simulink model "RelayZN_BlueRVO2_Control"  (R2023b)
settings: Solver=FixedStepAuto  StartTime=0.0  StopTime=600  FixedStep=0.01  RelTol=1e-3
values from neighbouring files (symbols this model uses):
  Kd_heave = 0.0666*Kc*Tc    (= 4.43668844611)    [RelayTest_controllerCalc.m]
  Kd_pitch = 0.0666*Kc*Tc    (= 1.01222543806)    [RelayTest_controllerCalc.m]
  Kd_roll = 0.0666*Kc*Tc    (= 0.877495471431)    [RelayTest_controllerCalc.m]
  Kd_surge = 0.0666*Kc*Tc    (= 11.6366264628)    [RelayTest_controllerCalc.m]
  Kd_sway = 0.0666*Kc*Tc    (= 3.84334224278)    [RelayTest_controllerCalc.m]
  Kd_yaw = 0.0666*Kc*Tc    (= 0.976135030348)    [RelayTest_controllerCalc.m]
  Ki_heave = 0.4*Kc/Tc    (= 0.123145727686)    [RelayTest_controllerCalc.m]
  Ki_pitch = 0.4*Kc/Tc    (= 0.865707662577)    [RelayTest_controllerCalc.m]
  Ki_roll = 0.4*Kc/Tc    (= 0.00801668103365)    [RelayTest_controllerCalc.m]
  Ki_surge = 0.4*Kc/Tc    (= 0.186852931714)    [RelayTest_controllerCalc.m]
  Ki_sway = 0.4*Kc/Tc    (= 0.0254608741636)    [RelayTest_controllerCalc.m]
  Ki_yaw = 0.4*Kc/Tc    (= 0.0110729266567)    [RelayTest_controllerCalc.m]
  Kp_heave = 0.2*Kc    (= 0.905736827128)    [RelayTest_controllerCalc.m]
  Kp_pitch = 0.2*Kc    (= 1.14706265291)    [RelayTest_controllerCalc.m]
  Kp_roll = 0.2*Kc    (= 0.102773850851)    [RelayTest_controllerCalc.m]
  Kp_surge = 0.2*Kc    (= 1.80686784967)    [RelayTest_controllerCalc.m]
  Kp_yaw = 0.2*Kc    (= 0.127394021185)    [RelayTest_controllerCalc.m]
libraries: slpidlib x18
(part 2 of 2)

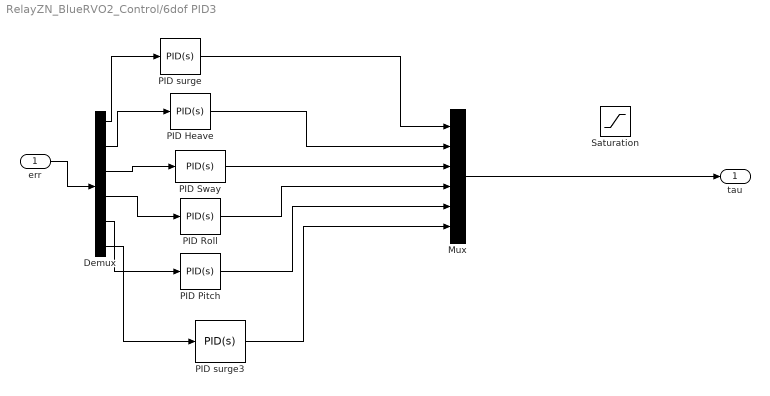
== system RelayZN_BlueRVO2_Control/6dof PID3 ==
  err : Inport
  Demux : Demux  Outputs=6
  Mux : Mux  Inputs=6
  PID Heave : slpidlib/PID Controller  Controller=PID  Form=Parallel  TimeDomain=Continuous-time  UseExternalTs=off  SampleTime=-1  IntegratorMethod=Forward Euler  FilterMethod=Forward Euler  ControllerParametersSource=internal  P=120  I=203  UseKiTs=off  D=17.7  N=100  UseFilter=on  TunerSelectOption=Transfer Function Based (PID Tuner App)  InitialConditionSource=internal  InitialConditionForIntegrator=0  InitialConditionForFilter=0  DifferentiatorICPrevScaledInput=0  ExternalReset=none  TrackingMode=off  Kt=1  LimitOutput=off  SatLimitsSource=internal  UpperSaturationLimit=inf  LowerSaturationLimit=-inf  LinearizeAsGain=on  AntiWindupMode=none  Kb=1  LimitIntegrator=off  UpperIntegratorSaturationLimit=inf  LowerIntegratorSaturationLimit=-inf  POutMin=[]  POutMax=[]  IOutMin=[]  IOutMax=[]  DOutMin=[]  DOutMax=[]  NOutMin=[]  NOutMax=[]  SumOutMin=[]  SumOutMax=[]  SaturationOutMin=[]  SaturationOutMax=[]  PParamMin=[]  PParamMax=[]  IParamMin=[]  IParamMax=[]  DParamMin=[]  DParamMax=[]  NParamMin=[]  NParamMax=[]  KbParamMin=[]  KbParamMax=[]  KtParamMin=[]  KtParamMax=[]  KbOutMin=[]  KbOutMax=[]  KtOutMin=[]  KtOutMax=[]  IntegratorOutMin=[]  IntegratorOutMax=[]  FilterOutMin=[]  FilterOutMax=[]  SumI1OutMin=[]  SumI1OutMax=[]  SumI2OutMin=[]  SumI2OutMax=[]  SumI3OutMin=[]  SumI3OutMax=[]  SumI4OutMin=[]  SumI4OutMax=[]  SumDOutMin=[]  SumDOutMax=[]  DifferentiatorOutMin=[]  DifferentiatorOutMax=[]  FilterDiffOutCoefMin=[]  FilterDiffOutCoefMax=[]  ReciprocalOutMin=[]  ReciprocalOutMax=[]  SumDenOutMin=[]  SumDenOutMax=[]  SumNumOutMin=[]  SumNumOutMax=[]  DivideOutMin=[]  DivideOutMax=[]  UdiffTsProdOutMin=[]  UdiffTsProdOutMax=[]  NTsProdOutMin=[]  NTsProdOutMax=[]  UintegralTsProdOutMin=[]  UintegralTsProdOutMax=[]  UngainTsProdOutMin=[]  UngainTsProdOutMax=[]  ClampingZeroOutDataTypeStr=Inherit: Inherit via back propagation  ClampingZeroOutMin=[]  ClampingZeroOutMax=[]  FilterDenConstantOutDataTypeStr=Inherit: Inherit via back propagation  FilterDenConstantOutMin=[]  FilterDenConstantOutMax=[]  PCopyOutDataTypeStr=Inherit: Inherit via back propagation  PCopyOutMin=[]  PCopyOutMax=[]  NCopyOutDataTypeStr=Inherit: Inherit via back propagation  NCopyOutMin=[]  NCopyOutMax=[]  IntegratorContinuousStateAttributes=''  IntegratorStateMustResolveToSignalObject=off  IntegratorRTWStateStorageClass=Auto  FilterContinuousStateAttributes=''  FilterStateMustResolveToSignalObject=off  FilterRTWStateStorageClass=Auto  ParallelPVariant=InternalParameters  IdealPVariant=Disabled  IVariant=InternalParameters  DVariant=InternalParameters  IntegratorVariant=Continuous  SatVariant=Disabled  AWVariant=Passthrough  PCopyVariant=Disabled  TRVariant=Disabled  FdbkBlocksVariant=Forward  IdealPFdbkVariant=Disabled  SatFdbkVariant=Disabled  DerivativeFilterVariant=ContFilter  NVariant=InternalParameters  NCopyVariant=Disabled  FilterICVariant=InternalICsFilter  IntegratorICVariant=InternalICs  ExternalResetVariant=Disabled  TRSumVariant=Passthrough  SumFdbkVariant=Disabled  SumVariant=Sum_PID  TsampFilterVariant=InternalTs  TsampNgainVariant=Passthrough  TsampIntegralVariant=Disabled_SignalSpec  ExternalSaturationOutDataTypeStr=Inherit: Same as second input
  PID Pitch : slpidlib/PID Controller  Controller=PID  Form=Parallel  TimeDomain=Continuous-time  UseExternalTs=off  SampleTime=-1  IntegratorMethod=Forward Euler  FilterMethod=Forward Euler  ControllerParametersSource=internal  P=4.2  I=8.4  UseKiTs=off  D=0.525  N=100  UseFilter=on  TunerSelectOption=Transfer Function Based (PID Tuner App)  InitialConditionSource=internal  InitialConditionForIntegrator=0  InitialConditionForFilter=0  DifferentiatorICPrevScaledInput=0  ExternalReset=none  TrackingMode=off  Kt=1  LimitOutput=off  SatLimitsSource=internal  UpperSaturationLimit=inf  LowerSaturationLimit=-inf  LinearizeAsGain=on  AntiWindupMode=none  Kb=1  LimitIntegrator=off  UpperIntegratorSaturationLimit=inf  LowerIntegratorSaturationLimit=-inf  POutMin=[]  POutMax=[]  IOutMin=[]  IOutMax=[]  DOutMin=[]  DOutMax=[]  NOutMin=[]  NOutMax=[]  SumOutMin=[]  SumOutMax=[]  SaturationOutMin=[]  SaturationOutMax=[]  PParamMin=[]  PParamMax=[]  IParamMin=[]  IParamMax=[]  DParamMin=[]  DParamMax=[]  NParamMin=[]  NParamMax=[]  KbParamMin=[]  KbParamMax=[]  KtParamMin=[]  KtParamMax=[]  KbOutMin=[]  KbOutMax=[]  KtOutMin=[]  KtOutMax=[]  IntegratorOutMin=[]  IntegratorOutMax=[]  FilterOutMin=[]  FilterOutMax=[]  SumI1OutMin=[]  SumI1OutMax=[]  SumI2OutMin=[]  SumI2OutMax=[]  SumI3OutMin=[]  SumI3OutMax=[]  SumI4OutMin=[]  SumI4OutMax=[]  SumDOutMin=[]  SumDOutMax=[]  DifferentiatorOutMin=[]  DifferentiatorOutMax=[]  FilterDiffOutCoefMin=[]  FilterDiffOutCoefMax=[]  ReciprocalOutMin=[]  ReciprocalOutMax=[]  SumDenOutMin=[]  SumDenOutMax=[]  SumNumOutMin=[]  SumNumOutMax=[]  DivideOutMin=[]  DivideOutMax=[]  UdiffTsProdOutMin=[]  UdiffTsProdOutMax=[]  NTsProdOutMin=[]  NTsProdOutMax=[]  UintegralTsProdOutMin=[]  UintegralTsProdOutMax=[]  UngainTsProdOutMin=[]  UngainTsProdOutMax=[]  ClampingZeroOutDataTypeStr=Inherit: Inherit via back propagation  ClampingZeroOutMin=[]  ClampingZeroOutMax=[]  FilterDenConstantOutDataTypeStr=Inherit: Inherit via back propagation  FilterDenConstantOutMin=[]  FilterDenConstantOutMax=[]  PCopyOutDataTypeStr=Inherit: Inherit via back propagation  PCopyOutMin=[]  PCopyOutMax=[]  NCopyOutDataTypeStr=Inherit: Inherit via back propagation  NCopyOutMin=[]  NCopyOutMax=[]  IntegratorContinuousStateAttributes=''  IntegratorStateMustResolveToSignalObject=off  IntegratorRTWStateStorageClass=Auto  FilterContinuousStateAttributes=''  FilterStateMustResolveToSignalObject=off  FilterRTWStateStorageClass=Auto  ParallelPVariant=InternalParameters  IdealPVariant=Disabled  IVariant=InternalParameters  DVariant=InternalParameters  IntegratorVariant=Continuous  SatVariant=Disabled  AWVariant=Passthrough  PCopyVariant=Disabled  TRVariant=Disabled  FdbkBlocksVariant=Forward  IdealPFdbkVariant=Disabled  SatFdbkVariant=Disabled  DerivativeFilterVariant=ContFilter  NVariant=InternalParameters  NCopyVariant=Disabled  FilterICVariant=InternalICsFilter  IntegratorICVariant=InternalICs  ExternalResetVariant=Disabled  TRSumVariant=Passthrough  SumFdbkVariant=Disabled  SumVariant=Sum_PID  TsampFilterVariant=InternalTs  TsampNgainVariant=Passthrough  TsampIntegralVariant=Disabled_SignalSpec  ExternalSaturationOutDataTypeStr=Inherit: Same as second input
  PID Roll : slpidlib/PID Controller  Controller=PID  Form=Parallel  TimeDomain=Continuous-time  UseExternalTs=off  SampleTime=-1  IntegratorMethod=Forward Euler  FilterMethod=Forward Euler  ControllerParametersSource=internal  P=3.6  I=6.37  UseKiTs=off  D=0.51  N=100  UseFilter=on  TunerSelectOption=Transfer Function Based (PID Tuner App)  InitialConditionSource=internal  InitialConditionForIntegrator=0  InitialConditionForFilter=0  DifferentiatorICPrevScaledInput=0  ExternalReset=none  TrackingMode=off  Kt=1  LimitOutput=off  SatLimitsSource=internal  UpperSaturationLimit=inf  LowerSaturationLimit=-inf  LinearizeAsGain=on  AntiWindupMode=none  Kb=1  LimitIntegrator=off  UpperIntegratorSaturationLimit=inf  LowerIntegratorSaturationLimit=-inf  POutMin=[]  POutMax=[]  IOutMin=[]  IOutMax=[]  DOutMin=[]  DOutMax=[]  NOutMin=[]  NOutMax=[]  SumOutMin=[]  SumOutMax=[]  SaturationOutMin=[]  SaturationOutMax=[]  PParamMin=[]  PParamMax=[]  IParamMin=[]  IParamMax=[]  DParamMin=[]  DParamMax=[]  NParamMin=[]  NParamMax=[]  KbParamMin=[]  KbParamMax=[]  KtParamMin=[]  KtParamMax=[]  KbOutMin=[]  KbOutMax=[]  KtOutMin=[]  KtOutMax=[]  IntegratorOutMin=[]  IntegratorOutMax=[]  FilterOutMin=[]  FilterOutMax=[]  SumI1OutMin=[]  SumI1OutMax=[]  SumI2OutMin=[]  SumI2OutMax=[]  SumI3OutMin=[]  SumI3OutMax=[]  SumI4OutMin=[]  SumI4OutMax=[]  SumDOutMin=[]  SumDOutMax=[]  DifferentiatorOutMin=[]  DifferentiatorOutMax=[]  FilterDiffOutCoefMin=[]  FilterDiffOutCoefMax=[]  ReciprocalOutMin=[]  ReciprocalOutMax=[]  SumDenOutMin=[]  SumDenOutMax=[]  SumNumOutMin=[]  SumNumOutMax=[]  DivideOutMin=[]  DivideOutMax=[]  UdiffTsProdOutMin=[]  UdiffTsProdOutMax=[]  NTsProdOutMin=[]  NTsProdOutMax=[]  UintegralTsProdOutMin=[]  UintegralTsProdOutMax=[]  UngainTsProdOutMin=[]  UngainTsProdOutMax=[]  ClampingZeroOutDataTypeStr=Inherit: Inherit via back propagation  ClampingZeroOutMin=[]  ClampingZeroOutMax=[]  FilterDenConstantOutDataTypeStr=Inherit: Inherit via back propagation  FilterDenConstantOutMin=[]  FilterDenConstantOutMax=[]  PCopyOutDataTypeStr=Inherit: Inherit via back propagation  PCopyOutMin=[]  PCopyOutMax=[]  NCopyOutDataTypeStr=Inherit: Inherit via back propagation  NCopyOutMin=[]  NCopyOutMax=[]  IntegratorContinuousStateAttributes=''  IntegratorStateMustResolveToSignalObject=off  IntegratorRTWStateStorageClass=Auto  FilterContinuousStateAttributes=''  FilterStateMustResolveToSignalObject=off  FilterRTWStateStorageClass=Auto  ParallelPVariant=InternalParameters  IdealPVariant=Disabled  IVariant=InternalParameters  DVariant=InternalParameters  IntegratorVariant=Continuous  SatVariant=Disabled  AWVariant=Passthrough  PCopyVariant=Disabled  TRVariant=Disabled  FdbkBlocksVariant=Forward  IdealPFdbkVariant=Disabled  SatFdbkVariant=Disabled  DerivativeFilterVariant=ContFilter  NVariant=InternalParameters  NCopyVariant=Disabled  FilterICVariant=InternalICsFilter  IntegratorICVariant=InternalICs  ExternalResetVariant=Disabled  TRSumVariant=Passthrough  SumFdbkVariant=Disabled  SumVariant=Sum_PID  TsampFilterVariant=InternalTs  TsampNgainVariant=Passthrough  TsampIntegralVariant=Disabled_SignalSpec  ExternalSaturationOutDataTypeStr=Inherit: Same as second input
  PID Sway : slpidlib/PID Controller  Controller=PID  Form=Parallel  TimeDomain=Continuous-time  UseExternalTs=off  SampleTime=-1  IntegratorMethod=Forward Euler  FilterMethod=Forward Euler  ControllerParametersSource=internal  P=120  I=208.7  UseKiTs=off  D=17.25  N=100  UseFilter=on  TunerSelectOption=Transfer Function Based (PID Tuner App)  InitialConditionSource=internal  InitialConditionForIntegrator=5  InitialConditionForFilter=0  DifferentiatorICPrevScaledInput=0  ExternalReset=none  TrackingMode=off  Kt=1  LimitOutput=off  SatLimitsSource=internal  UpperSaturationLimit=inf  LowerSaturationLimit=-inf  LinearizeAsGain=on  AntiWindupMode=none  Kb=1  LimitIntegrator=off  UpperIntegratorSaturationLimit=inf  LowerIntegratorSaturationLimit=-inf  POutMin=[]  POutMax=[]  IOutMin=[]  IOutMax=[]  DOutMin=[]  DOutMax=[]  NOutMin=[]  NOutMax=[]  SumOutMin=[]  SumOutMax=[]  SaturationOutMin=[]  SaturationOutMax=[]  PParamMin=[]  PParamMax=[]  IParamMin=[]  IParamMax=[]  DParamMin=[]  DParamMax=[]  NParamMin=[]  NParamMax=[]  KbParamMin=[]  KbParamMax=[]  KtParamMin=[]  KtParamMax=[]  KbOutMin=[]  KbOutMax=[]  KtOutMin=[]  KtOutMax=[]  IntegratorOutMin=[]  IntegratorOutMax=[]  FilterOutMin=[]  FilterOutMax=[]  SumI1OutMin=[]  SumI1OutMax=[]  SumI2OutMin=[]  SumI2OutMax=[]  SumI3OutMin=[]  SumI3OutMax=[]  SumI4OutMin=[]  SumI4OutMax=[]  SumDOutMin=[]  SumDOutMax=[]  DifferentiatorOutMin=[]  DifferentiatorOutMax=[]  FilterDiffOutCoefMin=[]  FilterDiffOutCoefMax=[]  ReciprocalOutMin=[]  ReciprocalOutMax=[]  SumDenOutMin=[]  SumDenOutMax=[]  SumNumOutMin=[]  SumNumOutMax=[]  DivideOutMin=[]  DivideOutMax=[]  UdiffTsProdOutMin=[]  UdiffTsProdOutMax=[]  NTsProdOutMin=[]  NTsProdOutMax=[]  UintegralTsProdOutMin=[]  UintegralTsProdOutMax=[]  UngainTsProdOutMin=[]  UngainTsProdOutMax=[]  ClampingZeroOutDataTypeStr=Inherit: Inherit via back propagation  ClampingZeroOutMin=[]  ClampingZeroOutMax=[]  FilterDenConstantOutDataTypeStr=Inherit: Inherit via back propagation  FilterDenConstantOutMin=[]  FilterDenConstantOutMax=[]  PCopyOutDataTypeStr=Inherit: Inherit via back propagation  PCopyOutMin=[]  PCopyOutMax=[]  NCopyOutDataTypeStr=Inherit: Inherit via back propagation  NCopyOutMin=[]  NCopyOutMax=[]  IntegratorContinuousStateAttributes=''  IntegratorStateMustResolveToSignalObject=off  IntegratorRTWStateStorageClass=Auto  FilterContinuousStateAttributes=''  FilterStateMustResolveToSignalObject=off  FilterRTWStateStorageClass=Auto  ParallelPVariant=InternalParameters  IdealPVariant=Disabled  IVariant=InternalParameters  DVariant=InternalParameters  IntegratorVariant=Continuous  SatVariant=Disabled  AWVariant=Passthrough  PCopyVariant=Disabled  TRVariant=Disabled  FdbkBlocksVariant=Forward  IdealPFdbkVariant=Disabled  SatFdbkVariant=Disabled  DerivativeFilterVariant=ContFilter  NVariant=InternalParameters  NCopyVariant=Disabled  FilterICVariant=InternalICsFilter  IntegratorICVariant=InternalICs  ExternalResetVariant=Disabled  TRSumVariant=Passthrough  SumFdbkVariant=Disabled  SumVariant=Sum_PID  TsampFilterVariant=InternalTs  TsampNgainVariant=Passthrough  TsampIntegralVariant=Disabled_SignalSpec  ExternalSaturationOutDataTypeStr=Inherit: Same as second input
  PID surge : slpidlib/PID Controller  Controller=PID  Form=Parallel  TimeDomain=Continuous-time  UseExternalTs=off  SampleTime=-1  IntegratorMethod=Forward Euler  FilterMethod=Forward Euler  ControllerParametersSource=internal  P=3.06  I=0.57  UseKiTs=off  D=4.1  N=100  UseFilter=on  TunerSelectOption=Transfer Function Based (PID Tuner App)  InitialConditionSource=internal  InitialConditionForIntegrator=0  InitialConditionForFilter=0  DifferentiatorICPrevScaledInput=0  ExternalReset=none  TrackingMode=off  Kt=1  LimitOutput=off  SatLimitsSource=internal  UpperSaturationLimit=inf  LowerSaturationLimit=-inf  LinearizeAsGain=on  AntiWindupMode=none  Kb=1  LimitIntegrator=off  UpperIntegratorSaturationLimit=inf  LowerIntegratorSaturationLimit=-inf  POutMin=[]  POutMax=[]  IOutMin=[]  IOutMax=[]  DOutMin=[]  DOutMax=[]  NOutMin=[]  NOutMax=[]  SumOutMin=[]  SumOutMax=[]  SaturationOutMin=[]  SaturationOutMax=[]  PParamMin=[]  PParamMax=[]  IParamMin=[]  IParamMax=[]  DParamMin=[]  DParamMax=[]  NParamMin=[]  NParamMax=[]  KbParamMin=[]  KbParamMax=[]  KtParamMin=[]  KtParamMax=[]  KbOutMin=[]  KbOutMax=[]  KtOutMin=[]  KtOutMax=[]  IntegratorOutMin=[]  IntegratorOutMax=[]  FilterOutMin=[]  FilterOutMax=[]  SumI1OutMin=[]  SumI1OutMax=[]  SumI2OutMin=[]  SumI2OutMax=[]  SumI3OutMin=[]  SumI3OutMax=[]  SumI4OutMin=[]  SumI4OutMax=[]  SumDOutMin=[]  SumDOutMax=[]  DifferentiatorOutMin=[]  DifferentiatorOutMax=[]  FilterDiffOutCoefMin=[]  FilterDiffOutCoefMax=[]  ReciprocalOutMin=[]  ReciprocalOutMax=[]  SumDenOutMin=[]  SumDenOutMax=[]  SumNumOutMin=[]  SumNumOutMax=[]  DivideOutMin=[]  DivideOutMax=[]  UdiffTsProdOutMin=[]  UdiffTsProdOutMax=[]  NTsProdOutMin=[]  NTsProdOutMax=[]  UintegralTsProdOutMin=[]  UintegralTsProdOutMax=[]  UngainTsProdOutMin=[]  UngainTsProdOutMax=[]  ClampingZeroOutDataTypeStr=Inherit: Inherit via back propagation  ClampingZeroOutMin=[]  ClampingZeroOutMax=[]  FilterDenConstantOutDataTypeStr=Inherit: Inherit via back propagation  FilterDenConstantOutMin=[]  FilterDenConstantOutMax=[]  PCopyOutDataTypeStr=Inherit: Inherit via back propagation  PCopyOutMin=[]  PCopyOutMax=[]  NCopyOutDataTypeStr=Inherit: Inherit via back propagation  NCopyOutMin=[]  NCopyOutMax=[]  IntegratorContinuousStateAttributes=''  IntegratorStateMustResolveToSignalObject=off  IntegratorRTWStateStorageClass=Auto  FilterContinuousStateAttributes=''  FilterStateMustResolveToSignalObject=off  FilterRTWStateStorageClass=Auto  ParallelPVariant=InternalParameters  IdealPVariant=Disabled  IVariant=InternalParameters  DVariant=InternalParameters  IntegratorVariant=Continuous  SatVariant=Disabled  AWVariant=Passthrough  PCopyVariant=Disabled  TRVariant=Disabled  FdbkBlocksVariant=Forward  IdealPFdbkVariant=Disabled  SatFdbkVariant=Disabled  DerivativeFilterVariant=ContFilter  NVariant=InternalParameters  NCopyVariant=Disabled  FilterICVariant=InternalICsFilter  IntegratorICVariant=InternalICs  ExternalResetVariant=Disabled  TRSumVariant=Passthrough  SumFdbkVariant=Disabled  SumVariant=Sum_PID  TsampFilterVariant=InternalTs  TsampNgainVariant=Passthrough  TsampIntegralVariant=Disabled_SignalSpec  ExternalSaturationOutDataTypeStr=Inherit: Same as second input
  PID surge3 : slpidlib/PID Controller  Controller=PID  Form=Parallel  TimeDomain=Continuous-time  UseExternalTs=off  SampleTime=-1  IntegratorMethod=Forward Euler  FilterMethod=Forward Euler  ControllerParametersSource=internal  P=3  I=6  UseKiTs=off  D=0.37  N=100  UseFilter=on  TunerSelectOption=Transfer Function Based (PID Tuner App)  InitialConditionSource=internal  InitialConditionForIntegrator=0  InitialConditionForFilter=0  DifferentiatorICPrevScaledInput=0  ExternalReset=none  TrackingMode=off  Kt=1  LimitOutput=off  SatLimitsSource=internal  UpperSaturationLimit=inf  LowerSaturationLimit=-inf  LinearizeAsGain=on  AntiWindupMode=none  Kb=1  LimitIntegrator=off  UpperIntegratorSaturationLimit=inf  LowerIntegratorSaturationLimit=-inf  POutMin=[]  POutMax=[]  IOutMin=[]  IOutMax=[]  DOutMin=[]  DOutMax=[]  NOutMin=[]  NOutMax=[]  SumOutMin=[]  SumOutMax=[]  SaturationOutMin=[]  SaturationOutMax=[]  PParamMin=[]  PParamMax=[]  IParamMin=[]  IParamMax=[]  DParamMin=[]  DParamMax=[]  NParamMin=[]  NParamMax=[]  KbParamMin=[]  KbParamMax=[]  KtParamMin=[]  KtParamMax=[]  KbOutMin=[]  KbOutMax=[]  KtOutMin=[]  KtOutMax=[]  IntegratorOutMin=[]  IntegratorOutMax=[]  FilterOutMin=[]  FilterOutMax=[]  SumI1OutMin=[]  SumI1OutMax=[]  SumI2OutMin=[]  SumI2OutMax=[]  SumI3OutMin=[]  SumI3OutMax=[]  SumI4OutMin=[]  SumI4OutMax=[]  SumDOutMin=[]  SumDOutMax=[]  DifferentiatorOutMin=[]  DifferentiatorOutMax=[]  FilterDiffOutCoefMin=[]  FilterDiffOutCoefMax=[]  ReciprocalOutMin=[]  ReciprocalOutMax=[]  SumDenOutMin=[]  SumDenOutMax=[]  SumNumOutMin=[]  SumNumOutMax=[]  DivideOutMin=[]  DivideOutMax=[]  UdiffTsProdOutMin=[]  UdiffTsProdOutMax=[]  NTsProdOutMin=[]  NTsProdOutMax=[]  UintegralTsProdOutMin=[]  UintegralTsProdOutMax=[]  UngainTsProdOutMin=[]  UngainTsProdOutMax=[]  ClampingZeroOutDataTypeStr=Inherit: Inherit via back propagation  ClampingZeroOutMin=[]  ClampingZeroOutMax=[]  FilterDenConstantOutDataTypeStr=Inherit: Inherit via back propagation  FilterDenConstantOutMin=[]  FilterDenConstantOutMax=[]  PCopyOutDataTypeStr=Inherit: Inherit via back propagation  PCopyOutMin=[]  PCopyOutMax=[]  NCopyOutDataTypeStr=Inherit: Inherit via back propagation  NCopyOutMin=[]  NCopyOutMax=[]  IntegratorContinuousStateAttributes=''  IntegratorStateMustResolveToSignalObject=off  IntegratorRTWStateStorageClass=Auto  FilterContinuousStateAttributes=''  FilterStateMustResolveToSignalObject=off  FilterRTWStateStorageClass=Auto  ParallelPVariant=InternalParameters  IdealPVariant=Disabled  IVariant=InternalParameters  DVariant=InternalParameters  IntegratorVariant=Continuous  SatVariant=Disabled  AWVariant=Passthrough  PCopyVariant=Disabled  TRVariant=Disabled  FdbkBlocksVariant=Forward  IdealPFdbkVariant=Disabled  SatFdbkVariant=Disabled  DerivativeFilterVariant=ContFilter  NVariant=InternalParameters  NCopyVariant=Disabled  FilterICVariant=InternalICsFilter  IntegratorICVariant=InternalICs  ExternalResetVariant=Disabled  TRSumVariant=Passthrough  SumFdbkVariant=Disabled  SumVariant=Sum_PID  TsampFilterVariant=InternalTs  TsampNgainVariant=Passthrough  TsampIntegralVariant=Disabled_SignalSpec  ExternalSaturationOutDataTypeStr=Inherit: Same as second input
  Saturation : Saturate  UpperLimit=16  LowerLimit=-16
  tau : Outport
  wires:
  Demux/6 -> PID surge3/1
  err/1 -> Demux/1
  Mux/1 -> tau/1
  Demux/1 -> PID surge/1
  Demux/3 -> PID Sway/1
  Demux/2 -> PID Heave/1
  Demux/4 -> PID Roll/1
  Demux/5 -> PID Pitch/1
  PID surge3/1 -> Mux/6
  PID surge/1 -> Mux/1
  PID Heave/1 -> Mux/2
  PID Sway/1 -> Mux/3
  PID Roll/1 -> Mux/4
  PID Pitch/1 -> Mux/5

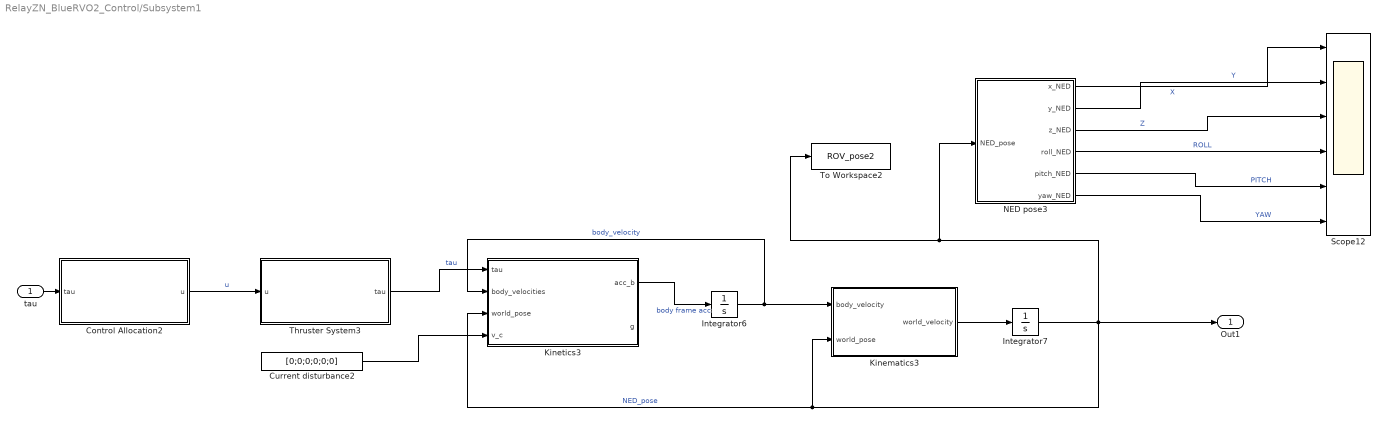
== system RelayZN_BlueRVO2_Control/Subsystem1 ==
  tau : Inport
  Control Allocation2 : MATLAB Function  TreatAsAtomicUnit=on
  Current disturbance2 : Constant  Value=[0;0;0;0;0;0]
  Integrator6 : Integrator  InitialCondition=[0;0;0;0;0;0]
  Integrator7 : Integrator  InitialCondition=[0;0;10;0;0;0]
  Kinematics3 : MATLAB Function  TreatAsAtomicUnit=on
  Kinetics3 : MATLAB Function  TreatAsAtomicUnit=on
  NED pose3 : MATLAB Function  TreatAsAtomicUnit=on
  Scope12 : Scope  NumInputPorts=6
  Thruster System3 : MATLAB Function  TreatAsAtomicUnit=on
  To Workspace2 : ToWorkspace  VariableName=ROV_pose2  SampleTime=-1
  Out1 : Outport
  wires:
  Integrator7/1 -> Out1/1, Kinetics3/3(world_pose), Kinematics3/2(world_pose), To Workspace2/1, NED pose3/1(NED_pose)  "NED_pose"
  Thruster System3/1(tau) -> Kinetics3/1(tau)  "tau"
  Integrator6/1 -> Kinetics3/2(body_velocities), Kinematics3/1(body_velocity)  "body_velocity"
  tau/1 -> Control Allocation2/1(tau)
  NED pose3/1(x_NED) -> Scope12/1  "X"
  Kinetics3/1(acc_b) -> Integrator6/1  "body frame acc"
  NED pose3/5(pitch_NED) -> Scope12/5  "PITCH"
  NED pose3/4(roll_NED) -> Scope12/4  "ROLL"
  Current disturbance2/1 -> Kinetics3/4(v_c)
  Control Allocation2/1(u) -> Thruster System3/1(u)  "u"
  Kinematics3/1(world_velocity) -> Integrator7/1
  NED pose3/6(yaw_NED) -> Scope12/6  "YAW"
  NED pose3/2(y_NED) -> Scope12/2  "Y"
  NED pose3/3(z_NED) -> Scope12/3  "Z"

== matlab function RelayZN_BlueRVO2_Control/Thruster System2 ==
  data: u input; tau output
function tau = fcn(u)
%The BlueROV2 heavy has an 8 thruster configuration: u is R^8.
%This function maps the PWM control input into generalised forces and
%moments of a 6 DoF with a specific 8 thruster configuration.


%Assuming linearity, the control force due to a thruster can be represented
%as F=Ku, with K is R^(8x8), diagonal. Using the BlueROV2 datasheed, the
%thrust coefficient matrix K is:
K=40*eye(8);

%We have to take into account the thrust configuration matrix (angle of
%each thruster with respect to the local XYZ (NED) frame attached 
%to the ROV:
T=[0.707    0.707   -0.707  -0.707      0       0     0     0;
   -0.707   0.707   -0.707   0.707      0       0     0     0;
      0        0        0       0      -1       1     1    -1;
    0.06    -0.06     0.06   -0.06  -0.218 -0.218 0.218  0.218;
    0.06     0.06    -0.06   -0.06   0.120 -0.120 0.120 -0.120;
  -0.1888  0.1888   0.1888  -0.1888    0      0     0      0];


tau = T*K*u;

== matlab function RelayZN_BlueRVO2_Control/inverse Kinematics1 ==
  data: error_NED input; error_body output; world_pose input
function error_body = fcn(error_NED,world_pose)

psi=world_pose(6);
theta=world_pose(5);
phi=world_pose(4);
%Getting the linear and angular velocites from body frame to NED world
%frame. The used orientation convention is Euler Angles -> Roll Pitch Yaw.
Rz=[cos(psi)  -sin(psi)  0;
    sin(psi)   cos(psi)  0;
       0           0     1];

Ry=[cos(theta)   0     sin(theta);
       0         1        0;
    -sin(theta)  0    cos(theta)];

Rx=[1      0          0;
    0   cos(phi)  -sin(phi);
    0   sin(phi)   cos(phi)];

R_bn=Rz*Ry*Rx;

T=[1 sin(phi)*tan(theta) cos(phi)*tan(theta);
   0        cos(phi)            -sin(phi);
   0 sin(phi)/cos(theta) cos(phi)*cos(theta)];

J=[R_bn         zeros([3,3]);
  zeros([3,3])          T];

 error_body= inv(J)*error_NED;

== matlab function RelayZN_BlueRVO2_Control/Subsystem1/Control Allocation2 ==
  data: tau input; u output
function u = fcn(tau)
%The BlueROV2 heavy has an 8 thruster configuration: u is R^8.
%This function maps the PWM control input into generalised forces and
%moments of a 6 DoF with a specific 8 thruster configuration.


%Assuming linearity, the control force due to a thruster can be represented
%as F=Ku, with K is R^(8x8), diagonal. Using the BlueROV2 datasheed, the
%thrust coefficient matrix K is:
K=40*eye(8);

%We have to take into account the thrust configuration matrix (angle of
%each thruster with respect to the local XYZ (NED) frame attached 
%to the ROV:
T=[0.707    0.707   -0.707  -0.707      0       0     0     0;
   -0.707   0.707   -0.707   0.707      0       0     0     0;
      0        0        0       0      -1       1     1    -1;
    0.06    -0.06     0.06   -0.06  -0.218 -0.218 0.218  0.218;
    0.06     0.06    -0.06   -0.06   0.120 -0.120 0.120 -0.120;
  -0.1888  0.1888   0.1888  -0.1888    0      0     0      0];


u = inv(K)*pinv(T)*tau;

== matlab function RelayZN_BlueRVO2_Control/Control Allocation2 ==
  data: tau input; u output
function u = fcn(tau)
%The BlueROV2 heavy has an 8 thruster configuration: u is R^8.
%This function maps the PWM control input into generalised forces and
%moments of a 6 DoF with a specific 8 thruster configuration.


%Assuming linearity, the control force due to a thruster can be represented
%as F=Ku, with K is R^(8x8), diagonal. Using the BlueROV2 datasheed, the
%thrust coefficient matrix K is:
K=40*eye(8);

%We have to take into account the thrust configuration matrix (angle of
%each thruster with respect to the local XYZ (NED) frame attached 
%to the ROV:
T=[0.707    0.707   -0.707  -0.707      0       0     0     0;
   -0.707   0.707   -0.707   0.707      0       0     0     0;
      0        0        0       0      -1       1     1    -1;
    0.06    -0.06     0.06   -0.06  -0.218 -0.218 0.218  0.218;
    0.06     0.06    -0.06   -0.06   0.120 -0.120 0.120 -0.120;
  -0.1888  0.1888   0.1888  -0.1888    0      0     0      0];


u = inv(K)*pinv(T)*tau;

== matlab function RelayZN_BlueRVO2_Control/Subsystem1/Kinematics3 ==
  data: body_velocity input; world_velocity output; world_pose input
function world_velocity = fcn(body_velocity,world_pose)

psi=world_pose(6);
theta=world_pose(5);
phi=world_pose(4);
%Getting the linear and angular velocites from body frame to NED world
%frame. The used orientation convention is Euler Angles -> Roll Pitch Yaw.
Rz=[cos(psi)  -sin(psi)  0;
    sin(psi)   cos(psi)  0;
       0           0     1];

Ry=[cos(theta)   0     sin(theta);
       0         1        0;
    -sin(theta)  0    cos(theta)];

Rx=[1      0          0;
    0   cos(phi)  -sin(phi);
    0   sin(phi)   cos(phi)];

R_bn=Rz*Ry*Rx;

T=[1 sin(phi)*tan(theta) cos(phi)*tan(theta);
   0        cos(phi)            -sin(phi);
   0 sin(phi)/cos(theta) cos(phi)*cos(theta)];

J=[R_bn         zeros([3,3]);
  zeros([3,3])          T];

world_velocity = J*body_velocity;

== matlab function RelayZN_BlueRVO2_Control/Subsystem1/Kinetics3 ==
  data: tau input; body_velocities input; world_pose input; acc_b output; v_c input; g output
function [acc_b, g] = fcn(tau,body_velocities,world_pose,v_c)
%The acceleration in body frame is determined 
%using the kinetic dynamic equations (Newton Euler):
%M_RB*dv + C_RB*v + M_A*dv_w + C_A*v_w + D*v_w + g = tau, where
%vw=v-v_c, where v_c is the speed of the waves - disturbances.

phi=world_pose(4);
theta=world_pose(5);
psi=world_pose(6);


u=body_velocities(1);
v=body_velocities(2);
w=body_velocities(3);
p=body_velocities(4);
q=body_velocities(5);
r=body_velocities(6);

%We shall first define some constants:
%ROV mass:
m=11.5;
%ROV weight
W=112.8;
%Buoyancy force
B=114.8;
%we place the centre of buoyancy in the center of the body frame:
rb=[0;0;0];
%position of the center of gravity w.r.t. the centre of buoyancy:
rg=[0;0;0.02];%in reality is 0.00019
%inertia moments about x,y,z in body frame are:
Ix=0.16; Iy=0.16; Iz=0.16;

%Added mass parameters:
X_du=-5.5; Y_dv=-12.7; Z_dw=-14.57; K_dp=-0.12; M_dq=-0.12; N_dr=-0.12;

%linear (e.g.X_u) and quadratic (e.g.X_u2 ->X_u|u|) dampig parameters:
X_u=-4.03; Y_v=-6.22; Z_w=-5.18; K_p=-0.07; M_q=-0.07; N_r=-0.07;
X_u2=-18.18; Y_v2=-21.66; Z_w2=-36.99; K_p2=-1.55; M_q2=-1.55; N_r2=-1.55;


M_RB =[m        0       0       0       m*rb(3)      0;
       0        m       0     -m*rb(3)    0          0;
       0        0       m       0         0          0;
       0      -m*rb(3)  0       Ix        0          0;
       m*rb(3)  0       0       0         Iy         0;
       0        0       0       0         0          Iz];
%u,v,w are linear velocities and p,q,r are angular velocities represented
%in body frame
C_RB =[0     0    0    0      m*w     0;
       0     0    0  -m*w      0      0;
       0     0    0   m*v    -m*u     0;
       0    m*w -m*v   0     Iz*r  -Iy*q;
     -m*w    0  -m*u -Iz*r     0    Ix*p;
      m*v  -m*u   0   Iy*q  -Ix*p     0]; 

% M_A = diag([X_du Y_dv Z_dw K_dp M_dq N_dr]);
% 
% C_A =[0     0       0       0     Z_dw*w       0;
%       0     0       0    -Z_dw*w     0       -X_du*u;
%       0     0       0    -Y_dv*v  X_du*u       0;
%       0   -Z_dw*w  Y_dv*v  0      -N_dr*r     M_dq*q;
%     Z_dw*w  0     -X_du*u N_dr*r    0        -K_dp*p;
%    -Y_dv*v X_du*u   0    -M_dq*q   K_dp*p      0];

%The Hydrodynamic damping can be approx with a linear damping D_L and a
%quadratic damping D_NL
D_L=-diag([X_u Y_v Z_w K_p M_q N_r]);

D_NL=-diag([X_u2*abs(u) Y_v2*abs(v) Z_w2*abs(w)...
           K_p2*abs(p) M_q2*abs(q) N_r2*abs(r)]);

D = D_L + D_NL;

%gravitational and
g = [(W-B)*sin(theta);
     -(W-B)*cos(theta)*sin(phi);
     -(W-B)*cos(theta)*cos(phi);
     rb(3)*W*cos(theta)*sin(phi);
     rb(3)*W*sin(theta);
     0];

%g = 0;

%with Ma and Ca
% acc_b=inv(M_RB+M_A)*(tau-C_RB*body_velocities ...
%                     -C_A*(body_velocities-v_c)-D*(body_velocities-v_c)-g);


%without Ma and Ca
acc_b=inv(M_RB)*(tau-C_RB*body_velocities-D*(body_velocities-v_c)-g);

== matlab function RelayZN_BlueRVO2_Control/Subsystem1/NED pose3 ==
  data: NED_pose input; x_NED output; y_NED output; z_NED output; roll_NED output; pitch_NED output; yaw_NED output
function [x_NED,y_NED,z_NED,roll_NED,pitch_NED,yaw_NED] = fcn(NED_pose)

x_NED =NED_pose(1);
y_NED =NED_pose(2);
z_NED =NED_pose(3);
roll_NED=NED_pose(4);
pitch_NED =NED_pose(5);
yaw_NED=NED_pose(6);

== matlab function RelayZN_BlueRVO2_Control/Subsystem1/Thruster System3 ==
  data: u input; tau output
function tau = fcn(u)
%The BlueROV2 heavy has an 8 thruster configuration: u is R^8.
%This function maps the PWM control input into generalised forces and
%moments of a 6 DoF with a specific 8 thruster configuration.


%Assuming linearity, the control force due to a thruster can be represented
%as F=Ku, with K is R^(8x8), diagonal. Using the BlueROV2 datasheed, the
%thrust coefficient matrix K is:
K=40*eye(8);

%We have to take into account the thrust configuration matrix (angle of
%each thruster with respect to the local XYZ (NED) frame attached 
%to the ROV:
T=[0.707    0.707   -0.707  -0.707      0       0     0     0;
   -0.707   0.707   -0.707   0.707      0       0     0     0;
      0        0        0       0      -1       1     1    -1;
    0.06    -0.06     0.06   -0.06  -0.218 -0.218 0.218  0.218;
    0.06     0.06    -0.06   -0.06   0.120 -0.120 0.120 -0.120;
  -0.1888  0.1888   0.1888  -0.1888    0      0     0      0];


tau = T*K*u;

== matlab function RelayZN_BlueRVO2_Control/inverse Kinematics3 ==
  data: error_NED input; error_body output; world_pose input
function error_body = fcn(error_NED,world_pose)

psi=world_pose(6);
theta=world_pose(5);
phi=world_pose(4);
%Getting the linear and angular velocites from body frame to NED world
%frame. The used orientation convention is Euler Angles -> Roll Pitch Yaw.
Rz=[cos(psi)  -sin(psi)  0;
    sin(psi)   cos(psi)  0;
       0           0     1];

Ry=[cos(theta)   0     sin(theta);
       0         1        0;
    -sin(theta)  0    cos(theta)];

Rx=[1      0          0;
    0   cos(phi)  -sin(phi);
    0   sin(phi)   cos(phi)];

R_bn=Rz*Ry*Rx;

T=[1 sin(phi)*tan(theta) cos(phi)*tan(theta);
   0        cos(phi)            -sin(phi);
   0 sin(phi)/cos(theta) cos(phi)*cos(theta)];

J=[R_bn         zeros([3,3]);
  zeros([3,3])          T];

 error_body= inv(J)*error_NED;

== matlab function RelayZN_BlueRVO2_Control/Kinematics1 ==
  data: body_velocity input; world_velocity output; world_pose input
function world_velocity = fcn(body_velocity,world_pose)

psi=world_pose(6);
theta=world_pose(5);
phi=world_pose(4);
%Getting the linear and angular velocites from body frame to NED world
%frame. The used orientation convention is Euler Angles -> Roll Pitch Yaw.
Rz=[cos(psi)  -sin(psi)  0;
    sin(psi)   cos(psi)  0;
       0           0     1];

Ry=[cos(theta)   0     sin(theta);
       0         1        0;
    -sin(theta)  0    cos(theta)];

Rx=[1      0          0;
    0   cos(phi)  -sin(phi);
    0   sin(phi)   cos(phi)];

R_bn=Rz*Ry*Rx;

T=[1 sin(phi)*tan(theta) cos(phi)*tan(theta);
   0        cos(phi)            -sin(phi);
   0 sin(phi)/cos(theta) cos(phi)*cos(theta)];

J=[R_bn         zeros([3,3]);
  zeros([3,3])          T];

world_velocity = J*body_velocity;

== matlab function RelayZN_BlueRVO2_Control/Kinetics1 ==
  data: tau input; body_velocities input; world_pose input; acc_b output; v_c input; g output
function [acc_b, g] = fcn(tau,body_velocities,world_pose,v_c)
%The acceleration in body frame is determined 
%using the kinetic dynamic equations (Newton Euler):
%M_RB*dv + C_RB*v + M_A*dv_w + C_A*v_w + D*v_w + g = tau, where
%vw=v-v_c, where v_c is the speed of the waves - disturbances.

phi=world_pose(4);
theta=world_pose(5);
psi=world_pose(6);


u=body_velocities(1);
v=body_velocities(2);
w=body_velocities(3);
p=body_velocities(4);
q=body_velocities(5);
r=body_velocities(6);

%We shall first define some constants:
%ROV mass:
m=11.5;
%ROV weight
W=112.8;
%Buoyancy force
B=114.8;
%we place the centre of buoyancy in the center of the body frame:
rb=[0;0;0];
%position of the center of gravity w.r.t. the centre of buoyancy:
rg=[0;0;0.02];%in reality is 0.00019
%inertia moments about x,y,z in body frame are:
Ix=0.16; Iy=0.16; Iz=0.16;

%Added mass parameters:
X_du=-5.5; Y_dv=-12.7; Z_dw=-14.57; K_dp=-0.12; M_dq=-0.12; N_dr=-0.12;

%linear (e.g.X_u) and quadratic (e.g.X_u2 ->X_u|u|) dampig parameters:
X_u=-4.03; Y_v=-6.22; Z_w=-5.18; K_p=-0.07; M_q=-0.07; N_r=-0.07;
X_u2=-18.18; Y_v2=-21.66; Z_w2=-36.99; K_p2=-1.55; M_q2=-1.55; N_r2=-1.55;


M_RB =[m        0       0       0       m*rb(3)      0;
       0        m       0     -m*rb(3)    0          0;
       0        0       m       0         0          0;
       0      -m*rb(3)  0       Ix        0          0;
       m*rb(3)  0       0       0         Iy         0;
       0        0       0       0         0          Iz];
%u,v,w are linear velocities and p,q,r are angular velocities represented
%in body frame
C_RB =[0     0    0    0      m*w     0;
       0     0    0  -m*w      0      0;
       0     0    0   m*v    -m*u     0;
       0    m*w -m*v   0     Iz*r  -Iy*q;
     -m*w    0  -m*u -Iz*r     0    Ix*p;
      m*v  -m*u   0   Iy*q  -Ix*p     0]; 

% M_A = diag([X_du Y_dv Z_dw K_dp M_dq N_dr]);
% 
% C_A =[0     0       0       0     Z_dw*w       0;
%       0     0       0    -Z_dw*w     0       -X_du*u;
%       0     0       0    -Y_dv*v  X_du*u       0;
%       0   -Z_dw*w  Y_dv*v  0      -N_dr*r     M_dq*q;
%     Z_dw*w  0     -X_du*u N_dr*r    0        -K_dp*p;
%    -Y_dv*v X_du*u   0    -M_dq*q   K_dp*p      0];

%The Hydrodynamic damping can be approx with a linear damping D_L and a
%quadratic damping D_NL
D_L=-diag([X_u Y_v Z_w K_p M_q N_r]);

D_NL=-diag([X_u2*abs(u) Y_v2*abs(v) Z_w2*abs(w)...
           K_p2*abs(p) M_q2*abs(q) N_r2*abs(r)]);

D = D_L + D_NL;

%gravitational and
g = [(W-B)*sin(theta);
     -(W-B)*cos(theta)*sin(phi);
     -(W-B)*cos(theta)*cos(phi);
     rb(3)*W*cos(theta)*sin(phi);
     rb(3)*W*sin(theta);
     0];

%g = 0;

%with Ma and Ca
% acc_b=inv(M_RB+M_A)*(tau-C_RB*body_velocities ...
%                     -C_A*(body_velocities-v_c)-D*(body_velocities-v_c)-g);


%without Ma and Ca
acc_b=inv(M_RB)*(tau-C_RB*body_velocities-D*(body_velocities-v_c)-g);

== matlab function RelayZN_BlueRVO2_Control/NED pose1 ==
  data: NED_pose input; x_NED output; y_NED output; z_NED output; roll_NED output; pitch_NED output; yaw_NED output
function [x_NED,y_NED,z_NED,roll_NED,pitch_NED,yaw_NED] = fcn(NED_pose)

x_NED =NED_pose(1);
y_NED =NED_pose(2);
z_NED =NED_pose(3);
roll_NED=NED_pose(4);
pitch_NED =NED_pose(5);
yaw_NED=NED_pose(6);

== matlab function RelayZN_BlueRVO2_Control/Thruster System1 ==
  data: u input; tau output
function tau = fcn(u)
%The BlueROV2 heavy has an 8 thruster configuration: u is R^8.
%This function maps the PWM control input into generalised forces and
%moments of a 6 DoF with a specific 8 thruster configuration.


%Assuming linearity, the control force due to a thruster can be represented
%as F=Ku, with K is R^(8x8), diagonal. Using the BlueROV2 datasheed, the
%thrust coefficient matrix K is:
K=40*eye(8);

%We have to take into account the thrust configuration matrix (angle of
%each thruster with respect to the local XYZ (NED) frame attached 
%to the ROV:
T=[0.707    0.707   -0.707  -0.707      0       0     0     0;
   -0.707   0.707   -0.707   0.707      0       0     0     0;
      0        0        0       0      -1       1     1    -1;
    0.06    -0.06     0.06   -0.06  -0.218 -0.218 0.218  0.218;
    0.06     0.06    -0.06   -0.06   0.120 -0.120 0.120 -0.120;
  -0.1888  0.1888   0.1888  -0.1888    0      0     0      0];


tau = T*K*u;

== matlab function RelayZN_BlueRVO2_Control/inverse Kinematics2 ==
  data: error_NED input; error_body output; world_pose input
function error_body = fcn(error_NED,world_pose)

psi=world_pose(6);
theta=world_pose(5);
phi=world_pose(4);
%Getting the linear and angular velocites from body frame to NED world
%frame. The used orientation convention is Euler Angles -> Roll Pitch Yaw.
Rz=[cos(psi)  -sin(psi)  0;
    sin(psi)   cos(psi)  0;
       0           0     1];

Ry=[cos(theta)   0     sin(theta);
       0         1        0;
    -sin(theta)  0    cos(theta)];

Rx=[1      0          0;
    0   cos(phi)  -sin(phi);
    0   sin(phi)   cos(phi)];

R_bn=Rz*Ry*Rx;

T=[1 sin(phi)*tan(theta) cos(phi)*tan(theta);
   0        cos(phi)            -sin(phi);
   0 sin(phi)/cos(theta) cos(phi)*cos(theta)];

J=[R_bn         zeros([3,3]);
  zeros([3,3])          T];

 error_body= inv(J)*error_NED;

== matlab function RelayZN_BlueRVO2_Control/Control Allocation1 ==
  data: tau input; u output
function u = fcn(tau)
%The BlueROV2 heavy has an 8 thruster configuration: u is R^8.
%This function maps the PWM control input into generalised forces and
%moments of a 6 DoF with a specific 8 thruster configuration.


%Assuming linearity, the control force due to a thruster can be represented
%as F=Ku, with K is R^(8x8), diagonal. Using the BlueROV2 datasheed, the
%thrust coefficient matrix K is:
K=40*eye(8);

%We have to take into account the thrust configuration matrix (angle of
%each thruster with respect to the local XYZ (NED) frame attached 
%to the ROV:
T=[0.707    0.707   -0.707  -0.707      0       0     0     0;
   -0.707   0.707   -0.707   0.707      0       0     0     0;
      0        0        0       0      -1       1     1    -1;
    0.06    -0.06     0.06   -0.06  -0.218 -0.218 0.218  0.218;
    0.06     0.06    -0.06   -0.06   0.120 -0.120 0.120 -0.120;
  -0.1888  0.1888   0.1888  -0.1888    0      0     0      0];


u = inv(K)*pinv(T)*tau;

== matlab function RelayZN_BlueRVO2_Control/Kinematics2 ==
  data: body_velocity input; world_velocity output; world_pose input
function world_velocity = fcn(body_velocity,world_pose)

psi=world_pose(6);
theta=world_pose(5);
phi=world_pose(4);
%Getting the linear and angular velocites from body frame to NED world
%frame. The used orientation convention is Euler Angles -> Roll Pitch Yaw.
Rz=[cos(psi)  -sin(psi)  0;
    sin(psi)   cos(psi)  0;
       0           0     1];

Ry=[cos(theta)   0     sin(theta);
       0         1        0;
    -sin(theta)  0    cos(theta)];

Rx=[1      0          0;
    0   cos(phi)  -sin(phi);
    0   sin(phi)   cos(phi)];

R_bn=Rz*Ry*Rx;

T=[1 sin(phi)*tan(theta) cos(phi)*tan(theta);
   0        cos(phi)            -sin(phi);
   0 sin(phi)/cos(theta) cos(phi)*cos(theta)];

J=[R_bn         zeros([3,3]);
  zeros([3,3])          T];

world_velocity = J*body_velocity;

== matlab function RelayZN_BlueRVO2_Control/Kinetics2 ==
  data: tau input; body_velocities input; world_pose input; acc_b output; v_c input; g output
function [acc_b, g] = fcn(tau,body_velocities,world_pose,v_c)
%The acceleration in body frame is determined 
%using the kinetic dynamic equations (Newton Euler):
%M_RB*dv + C_RB*v + M_A*dv_w + C_A*v_w + D*v_w + g = tau, where
%vw=v-v_c, where v_c is the speed of the waves - disturbances.

phi=world_pose(4);
theta=world_pose(5);
psi=world_pose(6);


u=body_velocities(1);
v=body_velocities(2);
w=body_velocities(3);
p=body_velocities(4);
q=body_velocities(5);
r=body_velocities(6);

%We shall first define some constants:
%ROV mass:
m=11.5;
%ROV weight
W=112.8;
%Buoyancy force
B=114.8;
%we place the centre of buoyancy in the center of the body frame:
rb=[0;0;0];
%position of the center of gravity w.r.t. the centre of buoyancy:
rg=[0;0;0.02];%in reality is 0.00019
%inertia moments about x,y,z in body frame are:
Ix=0.16; Iy=0.16; Iz=0.16;

%Added mass parameters:
X_du=-5.5; Y_dv=-12.7; Z_dw=-14.57; K_dp=-0.12; M_dq=-0.12; N_dr=-0.12;

%linear (e.g.X_u) and quadratic (e.g.X_u2 ->X_u|u|) dampig parameters:
X_u=-4.03; Y_v=-6.22; Z_w=-5.18; K_p=-0.07; M_q=-0.07; N_r=-0.07;
X_u2=-18.18; Y_v2=-21.66; Z_w2=-36.99; K_p2=-1.55; M_q2=-1.55; N_r2=-1.55;


M_RB =[m        0       0       0       m*rb(3)      0;
       0        m       0     -m*rb(3)    0          0;
       0        0       m       0         0          0;
       0      -m*rb(3)  0       Ix        0          0;
       m*rb(3)  0       0       0         Iy         0;
       0        0       0       0         0          Iz];
%u,v,w are linear velocities and p,q,r are angular velocities represented
%in body frame
C_RB =[0     0    0    0      m*w     0;
       0     0    0  -m*w      0      0;
       0     0    0   m*v    -m*u     0;
       0    m*w -m*v   0     Iz*r  -Iy*q;
     -m*w    0  -m*u -Iz*r     0    Ix*p;
      m*v  -m*u   0   Iy*q  -Ix*p     0]; 

% M_A = diag([X_du Y_dv Z_dw K_dp M_dq N_dr]);
% 
% C_A =[0     0       0       0     Z_dw*w       0;
%       0     0       0    -Z_dw*w     0       -X_du*u;
%       0     0       0    -Y_dv*v  X_du*u       0;
%       0   -Z_dw*w  Y_dv*v  0      -N_dr*r     M_dq*q;
%     Z_dw*w  0     -X_du*u N_dr*r    0        -K_dp*p;
%    -Y_dv*v X_du*u   0    -M_dq*q   K_dp*p      0];

%The Hydrodynamic damping can be approx with a linear damping D_L and a
%quadratic damping D_NL
D_L=-diag([X_u Y_v Z_w K_p M_q N_r]);

D_NL=-diag([X_u2*abs(u) Y_v2*abs(v) Z_w2*abs(w)...
           K_p2*abs(p) M_q2*abs(q) N_r2*abs(r)]);

D = D_L + D_NL;

%gravitational and
g = [(W-B)*sin(theta);
     -(W-B)*cos(theta)*sin(phi);
     -(W-B)*cos(theta)*cos(phi);
     rb(3)*W*cos(theta)*sin(phi);
     rb(3)*W*sin(theta);
     0];

%g = 0;

%with Ma and Ca
% acc_b=inv(M_RB+M_A)*(tau-C_RB*body_velocities ...
%                     -C_A*(body_velocities-v_c)-D*(body_velocities-v_c)-g);


%without Ma and Ca
acc_b=inv(M_RB)*(tau-C_RB*body_velocities-D*(body_velocities-v_c)-g);

== matlab function RelayZN_BlueRVO2_Control/NED pose2 ==
  data: NED_pose input; x_NED output; y_NED output; z_NED output; roll_NED output; pitch_NED output; yaw_NED output
function [x_NED,y_NED,z_NED,roll_NED,pitch_NED,yaw_NED] = fcn(NED_pose)

x_NED =NED_pose(1);
y_NED =NED_pose(2);
z_NED =NED_pose(3);
roll_NED=NED_pose(4);
pitch_NED =NED_pose(5);
yaw_NED=NED_pose(6);
